simulink model "eclipse_target_identification"  (Simulink 7.6)
settings: Solver=FixedStepDiscrete  StartTime=0.0  StopTime=inf  FixedStep=Ts  RelTol=1e-3
PreLoadFcn:
  | load_waypoints
values from neighbouring files (symbols this model uses):
  Ts = 0.009    [ident_template.m]
undefined symbols (not defined in the file or in its folder): DiscIntNeverNeededParam, g, mass, pitch_cmd2pitch, roll_cmd2roll, thrust_cmd2thrust, THRUST_CMD_GAIN, yaw_cmd2yaw
libraries: simulink x5, Hquad_control_LIB_SI x2, dspnetwork x2, powerlib_extras x1, idelinklib_tgtpref x1
settings Model: Creator=janosch  LastModifiedBy=burrimi  SimulationMode=external
settings DataIOCC: SaveOutput=off  SaveTime=off
settings OptimizationCC: OptimizeModelRefInitCode=on  LifeSpan=1
settings DebuggingCC: ParameterPrecisionLossMsg=none
settings HardwareCC: ProdIntDivRoundTo=Zero  ProdEndianess=LittleEndian  ProdHWDeviceType=Intel Pentium
settings RTWCC: SystemTargetFile=idelink_ert.tlc  GenerateMakefile=off  TemplateMakefile=idelink_ert.tmf  Description=Embedded IDE Link ERT  ProcessScript=idelink_ert_make_rtw_hook
settings CodeAppCC: IgnoreCustomStorageClasses=off
settings ERTFactory: TargetFcnLib=ansi_tfl_table_tmw.mat  TargetFunctionLibrary=ANSI_C  UtilityFuncGeneration=Auto  ERTMultiwordTypeDef=System defined  ERTCodeCoverageTool=None  ERTMultiwordLength=256  MultiwordLength=2048  GenerateFullHeader=on  GenerateSampleERTMain=off  GenerateTestInterfaces=off  IsPILTarget=off  ModelReferenceCompliant=on  ParMdlRefBuildCompliant=off  CompOptLevelCompliant=off  IncludeMdlTerminateFcn=on  GeneratePreprocessorConditionals=Disable all  CombineOutputUpdateFcns=on  CombineSignalStateStructs=off  SuppressErrorStatus=off  ERTFirstTimeCompliant=off  IncludeFileDelimiter=Auto  ERTCustomFileBanners=on  SupportAbsoluteTime=on  LogVarNameModifier=rt_  MatFileLogging=off  MultiInstanceERTCode=off  SupportNonFinite=on  SupportComplex=on  PurelyIntegerCode=off  SupportContinuousTime=off  SupportNonInlinedSFcns=on  SupportVariableSizeSignals=off  EnableShiftOperators=on  ParenthesesLevel=Nominal  PortableWordSizes=off  ModelStepFunctionPrototypeControlCompliant=on  CPPClassGenCompliant=off  AutosarCompliant=off  GenerateErtSFunction=off  CreateSILPILBlock=None  GenerateASAP2=off  ExtMode=on  ExtModeTransport=0  ExtModeStaticAlloc=off  ExtModeStaticAllocSize=1000000  ExtModeTesting=off  ExtModeMexFile=ext_comm  ExtModeIntrfLevel=Level1  InlinedParameterPlacement=Hierarchical  TargetOS=BareBoardExample  MultiInstanceErrorCode=Error  RateGroupingCode=on  RootIOFormat=Individual arguments  RTWCAPISignals=off  RTWCAPIParams=off  RTWCAPIStates=off  ERTSrcFileBannerTemplate=ert_code_template.cgt  ERTHdrFileBannerTemplate=ert_code_template.cgt  ERTDataSrcFileTemplate=ert_code_template.cgt  ERTDataHdrFileTemplate=ert_code_template.cgt  ERTCustomFileTemplate=example_file_process.tlc  CoverageDialogOpen=off  ModuleNamingRule=Unspecified  SignalDisplayLevel=10  ParamTuneLevel=10  GlobalDataDefinition=Auto  DataDefinitionFile=global.c  GlobalDataReference=Auto  ERTFilePackagingFormat=Modular  DataReferenceFile=global.h  GRTInterface=off  PreserveExpressionOrder=off  PreserveIfCondition=off  ConvertIfToSwitch=off  PreserveExternInFcnDecls=on  EnableUserReplacementTypes=off  MemSecPackage=--- None ---  MemSecDataConstants=Default  MemSecDataIO=Default  MemSecDataInternal=Default  MemSecDataParameters=Default  MemSecFuncInitTerm=Default  MemSecFuncExecute=Default  AdaptorName=Eclipse  exportIDEObj=on  ideObjName=IDE_Obj  oldideObjName=IDE_Obj  ideObjTimeout=50  oldideObjTimeout=50  ideObjBuildTimeout=1000  oldideObjBuildTimeout=1000  ProfileGenCode=off  profileBy=Tasks  ProfileNumSamples=100  InlineDSPBlks=off  projectOptions=Custom  debugCompilerOptions="-g -D\"_DEBUG\""  releaseCompilerOptions=-O2  getCompilerOptions=off  resetCompilerOptions=off  debugLinkerOptions=-lm  releaseLinkerOptions=-lm  customLinkerOptions=-lm  linkerOptionsStr=-lm  getLinkerOptions=off  resetLinkerOptions=off  systemStackSize=512  systemHeapSize=512  buildFormat=Project  buildAction=Build  overrunNotificationMethod=None  overrunNotificationFcn=myfunction  oldoverrunNotificationFcn=myfunction  configurePIL=off  configPILBlockAction=Create_PIL_block_build_and_download  DiagnosticActions=warning

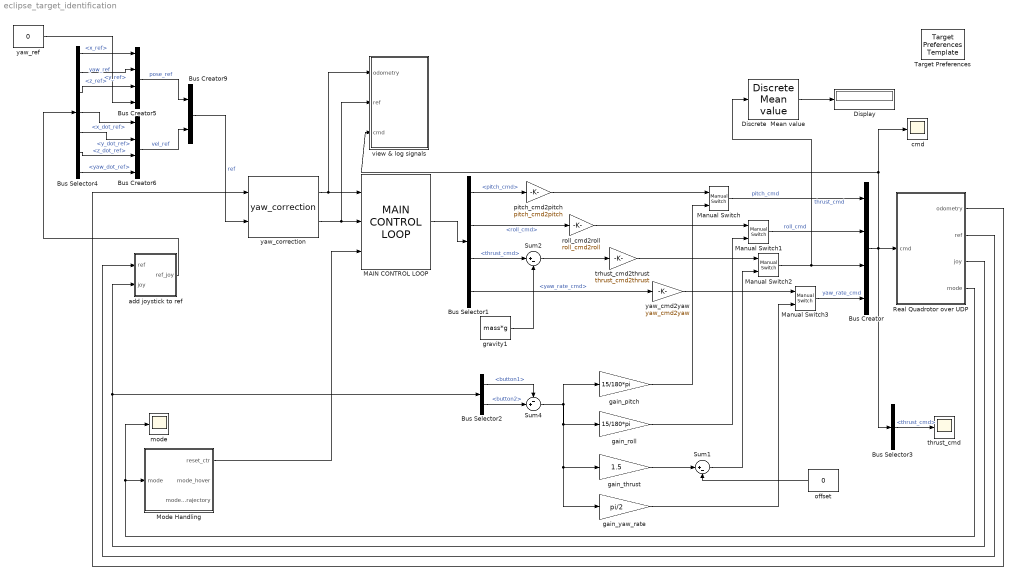
== system eclipse_target_identification ==
  Bus Creator : BusCreator
  Bus Creator5 : BusCreator
  Bus Creator6 : BusCreator
  Bus Creator9 : BusCreator  Inputs=2
  Bus Selector1 : BusSelector  OutputSignals=pitch_cmd,roll_cmd,thrust_cmd,yaw_rate_cmd
  Bus Selector2 : BusSelector  OutputSignals=joy_buttons.button1,joy_buttons.button2
  Bus Selector3 : BusSelector  OutputSignals=thrust_cmd
  Bus Selector4 : BusSelector  OutputSignals=pose_ref.x_ref,pose_ref.y_ref,pose_ref.z_ref,vel_ref.x_dot_ref,vel_ref.y_dot_ref,vel_ref.z_dot_ref,vel_ref.yaw_dot_ref
  Discrete  Mean value : powerlib_extras/Discrete Measurements/Discrete  Mean value  DialogController=POWERSYS.PowerSysDialog  SystemSampleTime=-1  Freq=1  Vinit=0  Ts=Ts
  Display : Display
  MAIN CONTROL LOOP : Hquad_control_LIB_SI/MAIN CONTROL LOOP  SystemSampleTime=-1
  Manual Switch{,1..3} (4 alike) : simulink/Signal Routing/Manual Switch  SystemSampleTime=-1  sw=1  action=0  varsize=off
  Mode Handling : Subsystem
  Real Quadrotor over UDP : Subsystem
  Sum1 : Sum  Inputs=|+-
  Sum2 : Sum  Inputs=|+-
  Sum4 : Sum  Inputs=-+|
  Target Preferences : idelinklib_tgtpref/Target Preferences Template  Tag=eclipseidetgtpref  SystemSampleTime=-1  library=off
  add joystick to ref : Subsystem
  cmd : Scope
      settings: TimeRange=10  YMin=-1  YMax=1  SaveName=ScopeData4
  gain_pitch : Gain  Gain=15/180*pi
  gain_roll : Gain  Gain=15/180*pi
  gain_thrust : Gain  Gain=1.5
  gain_yaw_rate : Gain  Gain=pi/2
  gravity1 : Constant  Value=mass*g
  mode : Scope
      settings: YMin=0  YMax=6  SaveName=ScopeData6
  offset : Constant  Value=0
  pitch_cmd2pitch : Gain  Gain=pitch_cmd2pitch
  roll_cmd2roll : Gain  Gain=roll_cmd2roll
  thrust_cmd : Scope
      settings: TimeRange=10  YMin=-1  YMax=1  SaveName=ScopeData9
  trhust_cmd2thrust : Gain  Gain=thrust_cmd2thrust
  view & log signals : Subsystem  AncestorBlock=Hquad_control_LIB_SI/view & log signals
  yaw_cmd2yaw : Gain  Gain=yaw_cmd2yaw
  yaw_correction : Hquad_control_LIB_SI/yaw_correction  SystemSampleTime=-1
  yaw_ref : Constant  Value=0
  wires:
  Real Quadrotor over UDP/3(joy) -> Bus Selector2/1, add joystick to ref/2(joy)
  Real Quadrotor over UDP/2(ref) -> add joystick to ref/1(ref)
  Real Quadrotor over UDP/4("mode   ") -> Mode Handling/1(mode), mode/1
  MAIN CONTROL LOOP/1 -> Bus Selector1/1
  yaw_correction/1 -> MAIN CONTROL LOOP/1, view & log signals/1(odometry)
  yaw_correction/2 -> MAIN CONTROL LOOP/2, view & log signals/2(ref)
  Real Quadrotor over UDP/1(odometry) -> yaw_correction/1
  Mode Handling/1(reset_ctr) -> MAIN CONTROL LOOP/3
  Bus Creator/1 -> Real Quadrotor over UDP/1(cmd), cmd/1, view & log signals/3(cmd), Bus Selector3/1
  Bus Selector2/2 -> Sum4/2  "<button2>"
  Bus Selector2/1 -> Sum4/1  "<button1>"
  Sum4/1 -> gain_pitch/1, gain_roll/1, gain_thrust/1, gain_yaw_rate/1
  Bus Selector3/1 -> thrust_cmd/1  "<thrust_cmd>"
  Manual Switch3/1 -> Bus Creator/4  "yaw_rate_cmd"
  Manual Switch2/1 -> Bus Creator/3, Discrete  Mean value/1  "thrust_cmd"
  Manual Switch/1 -> Bus Creator/1  "pitch_cmd"
  Manual Switch1/1 -> Bus Creator/2  "roll_cmd"
  Bus Selector1/1 -> pitch_cmd2pitch/1  "<pitch_cmd>"
  Bus Selector1/2 -> roll_cmd2roll/1  "<roll_cmd>"
  Bus Selector1/4 -> yaw_cmd2yaw/1  "<yaw_rate_cmd>"
  gain_pitch/1 -> Manual Switch/2
  gain_roll/1 -> Manual Switch1/2
  gain_yaw_rate/1 -> Manual Switch3/2
  pitch_cmd2pitch/1 -> Manual Switch/1
  roll_cmd2roll/1 -> Manual Switch1/1
  trhust_cmd2thrust/1 -> Manual Switch2/1
  yaw_cmd2yaw/1 -> Manual Switch3/1
  Sum2/1 -> trhust_cmd2thrust/1
  Bus Selector1/3 -> Sum2/1  "<thrust_cmd>"
  gravity1/1 -> Sum2/2
  Discrete  Mean value/1 -> Display/1
  Bus Creator9/1 -> yaw_correction/2  "ref"
  Bus Creator6/1 -> Bus Creator9/2  "vel_ref"
  Bus Creator5/1 -> Bus Creator9/1  "pose_ref"
  yaw_ref/1 -> Bus Creator5/4  "yaw_ref"
  add joystick to ref/1(ref_joy) -> Bus Selector4/1
  Bus Selector4/7 -> Bus Creator6/4  "<yaw_dot_ref>"
  Bus Selector4/6 -> Bus Creator6/3  "<z_dot_ref>"
  Bus Selector4/5 -> Bus Creator6/2  "<y_dot_ref>"
  Bus Selector4/4 -> Bus Creator6/1  "<x_dot_ref>"
  Bus Selector4/3 -> Bus Creator5/3  "<z_ref>"
  Bus Selector4/2 -> Bus Creator5/2  "<y_ref>"
  Bus Selector4/1 -> Bus Creator5/1  "<x_ref>"
  gain_thrust/1 -> Sum1/1
  Sum1/1 -> Manual Switch2/2
  offset/1 -> Sum1/2

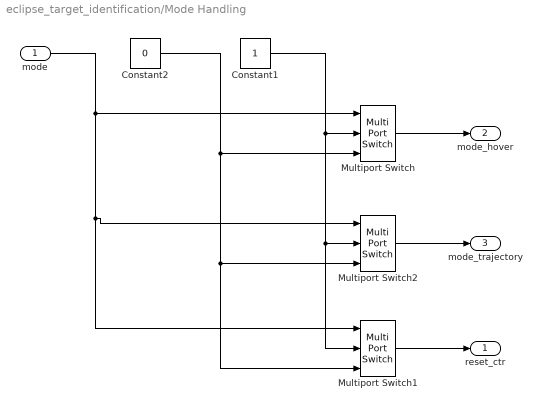
== system eclipse_target_identification/Mode Handling ==
  mode : Inport
  Constant1 : Constant
  Constant2 : Constant  Value=0
  Multiport Switch : MultiPortSwitch  DataPortOrder=Specify indices  Inputs=2  DataPortIndices={[1,2,3],0}  zeroidx=off
  Multiport Switch1 : MultiPortSwitch  DataPortOrder=Specify indices  Inputs=2  DataPortIndices={[10],0}  zeroidx=off
  Multiport Switch2 : MultiPortSwitch  DataPortOrder=Specify indices  Inputs=2  DataPortIndices={[4],0}  zeroidx=off
  reset_ctr : Outport
  mode_hover : Outport  Port=2
  mode_trajectory : Outport  Port=3
  wires:
  Constant1/1 -> Multiport Switch/2, Multiport Switch1/2, Multiport Switch2/2
  Constant2/1 -> Multiport Switch/3, Multiport Switch1/3, Multiport Switch2/3
  Multiport Switch1/1 -> reset_ctr/1
  mode/1 -> Multiport Switch/1, Multiport Switch1/1, Multiport Switch2/1
  Multiport Switch/1 -> mode_hover/1
  Multiport Switch2/1 -> mode_trajectory/1

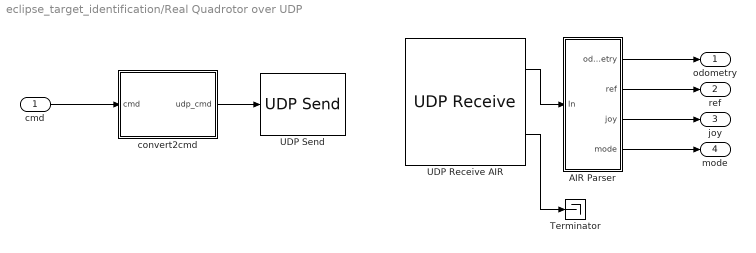
== system eclipse_target_identification/Real Quadrotor over UDP ==
  cmd : Inport
  AIR Parser : Subsystem
  Terminator : Terminator
  UDP Receive AIR : dspnetwork/UDP Receive  localURL='0.0.0.0'  localPort=9590  remoteURL='127.0.0.1'  remotePort=-1  recvBufferSize=8192  dims=30  signalDatatype=single  isVarSize=off  showBlockingTime=on  blockingTime=0.5  sampletime=Ts  blockPlatform=LINUX
  UDP Send : dspnetwork/UDP Send  remoteURL='127.0.0.1'  remotePort=9091  localURL='255.255.255.255'  localPortSource=Automatically determine  localPort=-1  sampletime=-1  blockPlatform=LINUX  separateLengthPort=0
  convert2cmd : Subsystem
  odometry : Outport
  ref : Outport  Port=2
  joy : Outport  Port=3
  "mode   " : Outport  Port=4  PortDimensions=1
  wires:
  UDP Receive AIR/2 -> Terminator/1
  AIR Parser/4(mode) -> "mode   "/1
  AIR Parser/3(joy) -> joy/1
  AIR Parser/2(ref) -> ref/1
  AIR Parser/1(odometry) -> odometry/1
  UDP Receive AIR/1 -> AIR Parser/1(In)
  convert2cmd/1(udp_cmd) -> UDP Send/1
  cmd/1 -> convert2cmd/1(cmd)

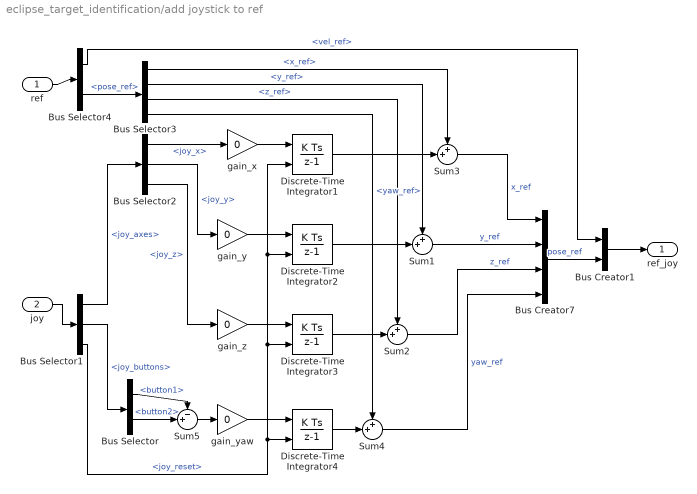
== system eclipse_target_identification/add joystick to ref ==
  ref : Inport
  joy : Inport  Port=2
  Bus Creator1 : BusCreator  Inputs=2
  Bus Creator7 : BusCreator
  Bus Selector : BusSelector  OutputSignals=button1,button2
  Bus Selector1 : BusSelector  OutputSignals=joy_axes,joy_buttons,joy_reset
  Bus Selector2 : BusSelector  OutputSignals=joy_x,joy_y,joy_z
  Bus Selector3 : BusSelector  OutputSignals=x_ref,y_ref,z_ref,yaw_ref
  Bus Selector4 : BusSelector  OutputSignals=vel_ref,pose_ref
  Discrete-Time Integrator{1..4} (4 alike) : DiscreteIntegrator  ExternalReset=rising  SampleTime=Ts  ICPrevOutput=DiscIntNeverNeededParam  ICPrevScaledInput=DiscIntNeverNeededParam
  Sum{1..4} (4 alike) : Sum  Inputs=++|
  Sum5 : Sum  Inputs=-+|
  gain_x : Gain  Gain=0
  gain_y : Gain  Gain=0
  gain_yaw : Gain  Gain=0
  gain_z : Gain  Gain=0
  ref_joy : Outport
  wires:
  Bus Selector2/1 -> gain_x/1  "<joy_x>"
  Bus Selector2/2 -> gain_y/1  "<joy_y>"
  Bus Selector2/3 -> gain_z/1  "<joy_z>"
  gain_x/1 -> Discrete-Time Integrator1/1
  gain_y/1 -> Discrete-Time Integrator2/1
  gain_z/1 -> Discrete-Time Integrator3/1
  Bus Selector3/1 -> Sum3/1  "<x_ref>"
  Bus Selector3/2 -> Sum1/1  "<y_ref>"
  Bus Selector3/3 -> Sum2/1  "<z_ref>"
  Discrete-Time Integrator1/1 -> Sum3/2
  Discrete-Time Integrator2/1 -> Sum1/2
  Discrete-Time Integrator3/1 -> Sum2/2
  Sum4/1 -> Bus Creator7/4  "yaw_ref"
  Sum2/1 -> Bus Creator7/3  "z_ref"
  Sum1/1 -> Bus Creator7/2  "y_ref"
  Sum3/1 -> Bus Creator7/1  "x_ref"
  Bus Selector1/2 -> Bus Selector/1  "<joy_buttons>"
  Bus Selector1/3 -> Discrete-Time Integrator3/2, Discrete-Time Integrator1/2, Discrete-Time Integrator2/2, Discrete-Time Integrator4/2  "<joy_reset>"
  Bus Selector/1 -> Sum5/1  "<button1>"
  Bus Selector/2 -> Sum5/2  "<button2>"
  Sum5/1 -> gain_yaw/1
  gain_yaw/1 -> Discrete-Time Integrator4/1
  Discrete-Time Integrator4/1 -> Sum4/2
  Bus Selector3/4 -> Sum4/1  "<yaw_ref>"
  joy/1 -> Bus Selector1/1
  Bus Selector1/1 -> Bus Selector2/1  "<joy_axes>"
  ref/1 -> Bus Selector4/1
  Bus Selector4/2 -> Bus Selector3/1  "<pose_ref>"
  Bus Selector4/1 -> Bus Creator1/1  "<vel_ref>"
  Bus Creator7/1 -> Bus Creator1/2  "pose_ref"
  Bus Creator1/1 -> ref_joy/1

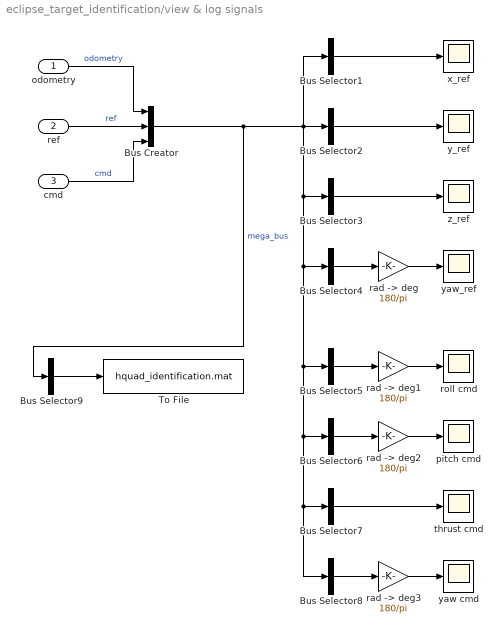
== system eclipse_target_identification/view & log signals ==
  odometry : Inport
  ref : Inport  Port=2
  cmd : Inport  Port=3
  Bus Creator : BusCreator  Inputs=3
  Bus Selector1 : BusSelector  OutputSignals=odometry.pos.x,odometry.vel.x_dot,ref.pose_ref.x_ref,ref.vel_ref.x_dot_ref  OutputAsBus=on
  Bus Selector2 : BusSelector  OutputSignals=odometry.pos.y,odometry.vel.y_dot,ref.pose_ref.y_ref,ref.vel_ref.y_dot_ref  OutputAsBus=on
  Bus Selector3 : BusSelector  OutputSignals=odometry.pos.z,odometry.vel.z_dot,ref.pose_ref.z_ref,ref.vel_ref.z_dot_ref  OutputAsBus=on
  Bus Selector4 : BusSelector  OutputSignals=odometry.rpy.yaw,odometry.ang_vel.ang_vel_z,ref.pose_ref.yaw_ref,ref.vel_ref.yaw_dot_ref  OutputAsBus=on
  Bus Selector5 : BusSelector  OutputSignals=odometry.rpy.roll,odometry.ang_vel.ang_vel_x,cmd.roll_cmd  OutputAsBus=on
  Bus Selector6 : BusSelector  OutputSignals=odometry.rpy.pitch,odometry.ang_vel.ang_vel_y,cmd.pitch_cmd  OutputAsBus=on
  Bus Selector7 : BusSelector  OutputSignals=odometry.pos.z,ref.pose_ref.z_ref,cmd.thrust_cmd  OutputAsBus=on
  Bus Selector8 : BusSelector  OutputSignals=odometry.rpy.yaw,odometry.ang_vel.ang_vel_z,cmd.yaw_rate_cmd  OutputAsBus=on
  Bus Selector9 : BusSelector  OutputSignals=odometry.pos.x,odometry.vel.x_dot,odometry.rpy.pitch,ref.pose_ref.x_ref,cmd.pitch_cmd,odometry.pos.y,odometry.vel.y_dot,odometry.rpy.roll,ref.pose_ref.y_ref,cmd.roll_cmd,odometry.pos.z,odometry.vel.z_dot,ref.pose_ref.z_ref,cmd.thrust_cmd,odometry.rpy.yaw,odometry.ang_vel.ang_vel_z,ref.pose_ref.yaw_ref,cmd.yaw_rate_cmd  OutputAsBus=on
  To File : ToFile  Filename=hquad_identification.mat  MatrixName=hquad_identification
  pitch cmd : Scope
      settings: YMin=-15  YMax=15  SaveName=ScopeData2
  rad -> deg{,1..3} (4 alike) : Gain  Gain=180/pi
  roll cmd : Scope
      settings: YMin=-100  YMax=100
  thrust cmd : Scope
      settings: YMin=-3  YMax=3  SaveName=ScopeData11
  x_ref : Scope
      settings: TimeRange=40  YMin=-1.5  YMax=1.5  SaveName=ScopeData3
  y_ref : Scope
      settings: TimeRange=40  YMin=-1.5  YMax=1.5
  yaw cmd : Scope
      settings: YMin=-60  YMax=-0  SaveName=ScopeData10
  yaw_ref : Scope
      settings: TimeRange=39.996  YMin=0  YMax=3250  SaveName=ScopeData8
  z_ref : Scope
      settings: YMin=-0.05  YMax=1.05  SaveName=ScopeData5
  wires:
  Bus Selector9/1 -> To File/1
  "rad -> deg"/1 -> yaw_ref/1
  "rad -> deg1"/1 -> roll cmd/1
  "rad -> deg2"/1 -> pitch cmd/1
  "rad -> deg3"/1 -> yaw cmd/1
  odometry/1 -> Bus Creator/1  "odometry"
  ref/1 -> Bus Creator/2  "ref"
  cmd/1 -> Bus Creator/3  "cmd"
  Bus Creator/1 -> Bus Selector9/1, Bus Selector1/1, Bus Selector2/1, Bus Selector3/1, Bus Selector4/1, Bus Selector5/1, Bus Selector6/1, Bus Selector7/1, Bus Selector8/1  "mega_bus"
  Bus Selector1/1 -> x_ref/1
  Bus Selector2/1 -> y_ref/1
  Bus Selector3/1 -> z_ref/1
  Bus Selector4/1 -> "rad -> deg"/1
  Bus Selector7/1 -> thrust cmd/1
  Bus Selector5/1 -> "rad -> deg1"/1
  Bus Selector6/1 -> "rad -> deg2"/1
  Bus Selector8/1 -> "rad -> deg3"/1

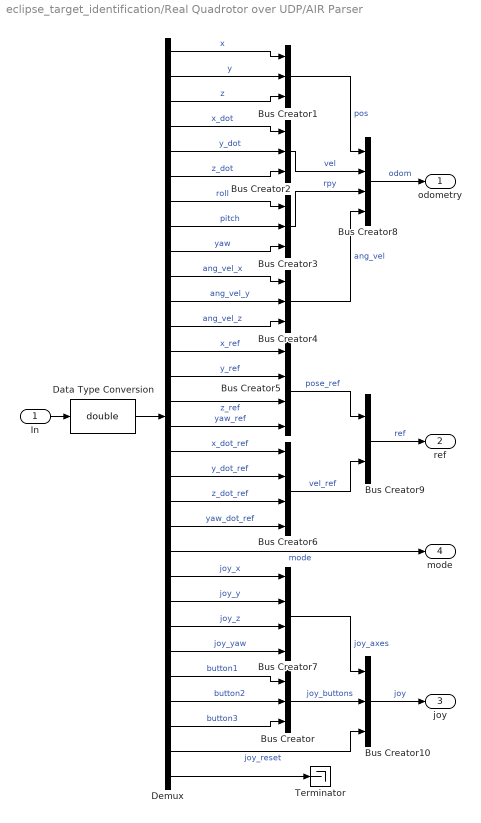
== system eclipse_target_identification/Real Quadrotor over UDP/AIR Parser ==
  In : Inport
  Bus Creator{,1..4,10} (6 alike) : BusCreator  Inputs=3
  Bus Creator{5..8} (4 alike) : BusCreator
  Bus Creator9 : BusCreator  Inputs=2
  Data Type Conversion : DataTypeConversion  OutDataTypeStr=double
  Demux : Demux  Outputs=30
  Terminator : Terminator
  odometry : Outport
  ref : Outport  Port=2
  joy : Outport  Port=3
  mode : Outport  Port=4
  wires:
  Demux/30 -> Terminator/1
  Bus Creator8/1 -> odometry/1  "odom"
  Bus Creator9/1 -> ref/1  "ref"
  Bus Creator10/1 -> joy/1  "joy"
  Demux/29 -> Bus Creator10/3  "joy_reset"
  Bus Creator1/1 -> Bus Creator8/1  "pos"
  Bus Creator2/1 -> Bus Creator8/2  "vel"
  Bus Creator3/1 -> Bus Creator8/3  "rpy"
  Bus Creator4/1 -> Bus Creator8/4  "ang_vel"
  Bus Creator/1 -> Bus Creator10/2  "joy_buttons"
  Demux/27 -> Bus Creator/2  "button2"
  Demux/28 -> Bus Creator/3  "button3"
  Demux/26 -> Bus Creator/1  "button1"
  Bus Creator7/1 -> Bus Creator10/1  "joy_axes"
  Demux/25 -> Bus Creator7/4  "joy_yaw"
  Demux/24 -> Bus Creator7/3  "joy_z"
  Demux/23 -> Bus Creator7/2  "joy_y"
  Demux/22 -> Bus Creator7/1  "joy_x"
  Bus Creator6/1 -> Bus Creator9/2  "vel_ref"
  Bus Creator5/1 -> Bus Creator9/1  "pose_ref"
  Demux/21 -> mode/1  "mode"
  Demux/10 -> Bus Creator4/1  "ang_vel_x"
  Demux/11 -> Bus Creator4/2  "ang_vel_y"
  Demux/12 -> Bus Creator4/3  "ang_vel_z"
  Demux/20 -> Bus Creator6/4  "yaw_dot_ref"
  Demux/17 -> Bus Creator6/1  "x_dot_ref"
  Demux/18 -> Bus Creator6/2  "y_dot_ref"
  Demux/19 -> Bus Creator6/3  "z_dot_ref"
  Demux/6 -> Bus Creator2/3  "z_dot"
  Demux/5 -> Bus Creator2/2  "y_dot"
  Demux/4 -> Bus Creator2/1  "x_dot"
  Demux/3 -> Bus Creator1/3  "z"
  Demux/2 -> Bus Creator1/2  "y"
  Demux/16 -> Bus Creator5/4  "yaw_ref"
  Demux/13 -> Bus Creator5/1  "x_ref"
  Demux/14 -> Bus Creator5/2  "y_ref"
  Demux/15 -> Bus Creator5/3  "z_ref"
  Demux/9 -> Bus Creator3/3  "yaw"
  Demux/8 -> Bus Creator3/2  "pitch"
  Demux/7 -> Bus Creator3/1  "roll"
  Demux/1 -> Bus Creator1/1  "x"
  Data Type Conversion/1 -> Demux/1
  In/1 -> Data Type Conversion/1

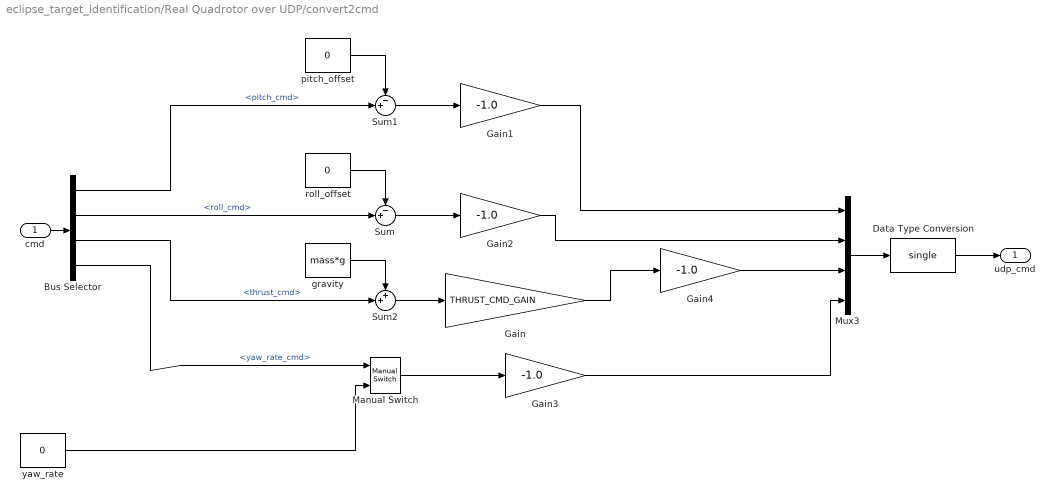
== system eclipse_target_identification/Real Quadrotor over UDP/convert2cmd ==
  cmd : Inport
  Bus Selector : BusSelector  OutputSignals=pitch_cmd,roll_cmd,thrust_cmd,yaw_rate_cmd
  Data Type Conversion : DataTypeConversion  OutDataTypeStr=single
  Gain : Gain  Gain=THRUST_CMD_GAIN
  Gain{1..4} (4 alike) : Gain  Gain=-1.0
  Manual Switch : simulink/Signal Routing/Manual Switch  SystemSampleTime=-1  sw=1  action=0  varsize=off
  Mux3 : Mux
  Sum : Sum  Inputs=-+|
  Sum1 : Sum  Inputs=-+|
  Sum2 : Sum  Inputs=++|
  gravity : Constant  Value=mass*g
  pitch_offset : Constant  Value=0
  roll_offset : Constant  Value=0
  yaw_rate : Constant  Value=0
  udp_cmd : Outport
  wires:
  Bus Selector/2 -> Sum/2  "<roll_cmd>"
  Bus Selector/1 -> Sum1/2  "<pitch_cmd>"
  Bus Selector/4 -> Manual Switch/1  "<yaw_rate_cmd>"
  Bus Selector/3 -> Sum2/2  "<thrust_cmd>"
  cmd/1 -> Bus Selector/1
  yaw_rate/1 -> Manual Switch/2
  Manual Switch/1 -> Gain3/1
  Sum2/1 -> Gain/1
  gravity/1 -> Sum2/1
  Data Type Conversion/1 -> udp_cmd/1
  Mux3/1 -> Data Type Conversion/1
  Sum/1 -> Gain2/1
  Sum1/1 -> Gain1/1
  pitch_offset/1 -> Sum1/1
  Gain1/1 -> Mux3/1
  Gain/1 -> Gain4/1
  roll_offset/1 -> Sum/1
  Gain2/1 -> Mux3/2
  Gain3/1 -> Mux3/4
  Gain4/1 -> Mux3/3
